simulink model "TP_Sim"  (R2024b)
settings: Solver=ode45  StartTime=0.0  StopTime=30  RelTol=1e-3
settings Model: Creator=user  LastModifiedBy=user

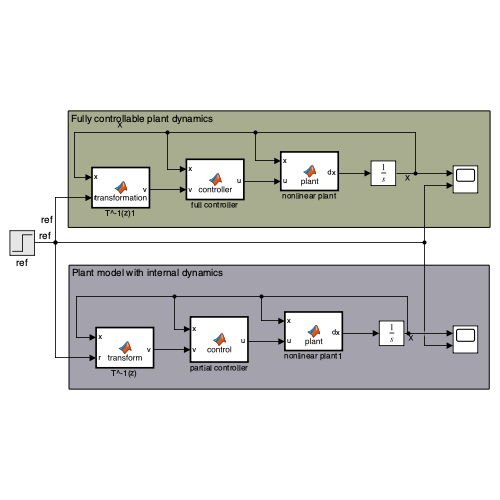
[thumbnail: Simulink's stored preview of the top-level diagram]
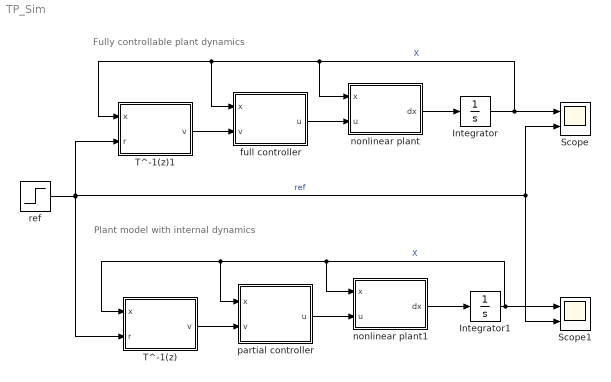
== system TP_Sim ==
  note: Plant model with internal dynamics
  note: Fully controllable plant dynamics
  Integrator : Integrator  InitialCondition=[1, 0.5, 0.4]'  ZeroCross=off
  Integrator1 : Integrator  InitialCondition=[.1, 0.5, 0.04]'  ZeroCross=off
  Scope : Scope  NumInputPorts=2
  Scope1 : Scope  NumInputPorts=2
  T^-1(z) : MATLAB Function  TreatAsAtomicUnit=on
  T^-1(z)1 : MATLAB Function  TreatAsAtomicUnit=on
  full controller : MATLAB Function  TreatAsAtomicUnit=on
  nonlinear plant : MATLAB Function  TreatAsAtomicUnit=on
  nonlinear plant1 : MATLAB Function  TreatAsAtomicUnit=on
  partial controller : MATLAB Function  TreatAsAtomicUnit=on
  ref : Step  Time=10  Before=1  After=2  SampleTime=0
  wires:
  ref/1 -> T^-1(z)1/2(r), Scope/2, Scope1/2, T^-1(z)/2(r)  "ref"
  Integrator/1 -> full controller/1(x), T^-1(z)1/1(x), nonlinear plant/1(x), Scope/1  "X"
  nonlinear plant/1(dx) -> Integrator/1
  full controller/1(u) -> nonlinear plant/2(u)
  Integrator1/1 -> Scope1/1, nonlinear plant1/1(x), partial controller/1(x), T^-1(z)/1(x)  "X"
  nonlinear plant1/1(dx) -> Integrator1/1
  partial controller/1(u) -> nonlinear plant1/2(u)
  T^-1(z)/1(v) -> partial controller/2(v)
  T^-1(z)1/1(v) -> full controller/2(v)

== matlab function TP_Sim/full controller ==
  data: x input; v input; u output
function u = controller(x,v)
a = 1; k = 0.4; m = 2;
u = (v + a*x(3)*x(2)/(m*x(1)) + k*x(2)/m)*(m*x(1))/(x(3));

== matlab function TP_Sim/nonlinear plant ==
  data: x input; u input; dx output
function dx = plant(x,u)
dx = zeros(3,1);
a = 1; k = 0.4; m = 2;
dx(1) = x(2);
dx(2) = (a*x(3)-k*x(1))/m;
dx(3) = -(x(3)/x(1))*(x(2)-u/a);

== matlab function TP_Sim/partial controller ==
  data: x input; v input; u output
function u = control(x, v)
a = 1; k = 0.4; m = 2; %K = 2;

u = (m*x(1)/x(3))*(v + a*x(3)*x(2)/(m*x(1))+k*x(2)/m);

== matlab function TP_Sim/nonlinear plant1 ==
  data: x input; u input; dx output
function dx = plant(x,u)
dx = zeros(3,1);
a = 1; k = 0.4; m = 2;
dx(1) = x(2);
dx(2) = (a*x(3)-k*x(1))/m;
dx(3) = -(x(3)/x(1))*(x(2)-u/a);

== matlab function TP_Sim/T^-1(z) ==
  data: x input; v output; r input; K2 parameter
function v = transform(x, r, K2)
a = 1; m = 2; k = 0.4;
z1 = x(2);
z2 = (a*x(3)-k*x(1))/m;
v = K2(1)*(r-z1)-K2(2)*z2;

== matlab function TP_Sim/T^-1(z)1 ==
  data: x input; v output; r input; K parameter
function v = transformation(x, r, K)
a = 1; m = 2; k = 0.4;
z1 = x(1);
z2 = x(2);
z3 = (a*x(3)-k*x(1))/m;
v = K(1)*(r-z1)-K(2)*z2 - K(3)*z3;
